simulink model "stmnucleo_I2C_temp_extendedMode"  (R2022a)
settings: Solver=FixedStepAuto  StartTime=0.0  StopTime=30  RelTol=1e-3  EnableMultiTasking=on
libraries: hdlsllib x4, simulink x4, mbedblockslib x4
settings Model: SimulationMode=external  ExtModeTrigDuration=10  Creator=The MathWorks, Inc.  LastModifiedBy=FUGAZI
settings SolverCC: AlgebraicLoopSolver=TrustRegion  MaxZcPerStep=1
settings DataIOCC: LimitDataPoints=on  ReturnWorkspaceOutputs=off
settings OptimizationCC: BlockReduction=off  LifeSpan=Inf  MaxStackSize=64
settings DebuggingCC: UnconnectedInputMsg=warning  UnconnectedOutputMsg=warning  UnconnectedLineMsg=warning  AllowSymbolicDim=off  SFUnexpectedBacktrackingDiag=warning  SFNoUnconditionalDefaultTransitionDiag=warning  SFExecutionAtInitializationDiag=none  SFMachineParentedDataDiag=warning  ArithmeticOperatorsInVariantConditions=warning
settings HardwareCC: ProdBitPerPointer=32  ProdBitPerSizeT=32  ProdBitPerPtrDiffT=32  ProdLargestAtomicInteger=Long  ProdLargestAtomicFloat=Double  ProdWordSize=32  ProdLongLongMode=on  ProdHWDeviceType=ARM Compatible->ARM Cortex
settings ModelReferenceCC: PropagateSignalLabelsOutOfModel=off
settings SFSimCC: SimUseLocalCustomCode=off
settings RTWCC: SystemTargetFile=ert.tlc  HardwareBoard=STM32 Nucleo L476RG  TemplateMakefile=ert_default_tmf  RTWUseLocalCustomCode=off  Toolchain=GNU Tools for ARM Embedded Processors  BuildConfiguration=Faster Runs  DLArmComputeVersion=19.05
settings CodeAppCC: StateflowObjectComments=on
settings ERTTargetCC: CodeReplacementLibrary=ARM Cortex-M (Optimized)  MultiwordLength=2048  ERTCustomFileBanners=off  SupportContinuousTime=on  SupportNonInlinedSFcns=on  RemoveResetFunc=off  ModelStepFunctionPrototypeControlCompliant=off  ExtModeTransport=3  ExtModeStaticAlloc=on  ExtModeStaticAllocSize=2000  ExtModeMexFile=ext_xcp  ExtModeIntrfLevel=Level2 - Open  ConvertIfToSwitch=off  SuppressUnreachableDefaultCases=off
settings ConfigComp: CovMetricSettings=dw  CovSaveCumulativeToWorkspaceVar=on  CovSaveSingleToWorkspaceVar=on  CovExternalEMLEnable=off

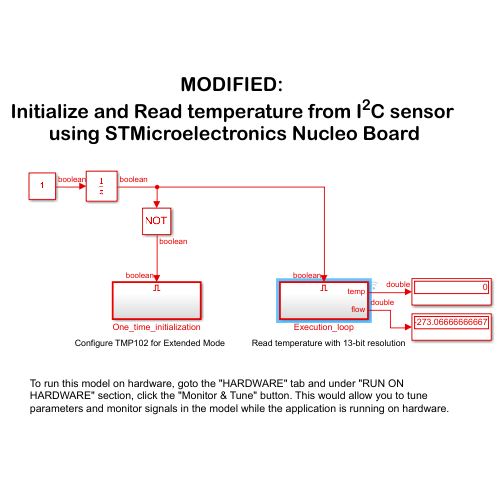
[thumbnail: Simulink's stored preview of the top-level diagram]
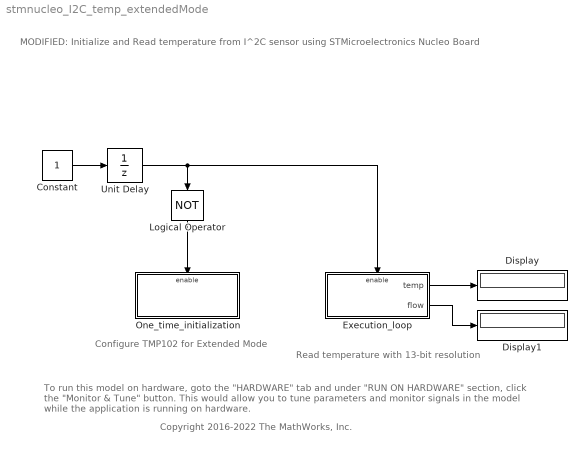
== system stmnucleo_I2C_temp_extendedMode ==
  note: Read temperature with 13-bit resolution
  note: Configure TMP102 for Extended Mode
  note: Copyright 2016-2022 The MathWorks, Inc.
  note: MODIFIED:
      | Initialize and Read temperature from I^2C sensor
      |  using STMicroelectronics Nucleo Board
  note: To run this model on hardware, goto the "HARDWARE" tab and under "RUN ON HARDWARE" section, click the "Monitor & Tune" button. This would allow you to tune parameters and monitor signals in the model while the application is running on hardware.
  Constant : Constant  OutDataTypeStr=boolean  SampleTime=0.1
  Display : Display
      settings: Format=hex (Stored Integer)
  Display1 : Display
      settings: Format=hex (Stored Integer)
  Execution_loop : Subsystem  TreatAsAtomicUnit=on
  Logical Operator : Logic  Operator=NOT  AllPortsSameDT=off  OutDataTypeStr=boolean
  One_time_initialization : Subsystem  TreatAsAtomicUnit=on
  Unit Delay : UnitDelay  SampleTime=-1  HasFrameUpgradeWarning=on
  wires:
  Constant/1 -> Unit Delay/1
  Unit Delay/1 -> Execution_loop/Enable, Logical Operator/1
  Logical Operator/1 -> One_time_initialization/Enable
  Execution_loop/1(temp) -> Display/1
  Execution_loop/2(flow) -> Display1/1

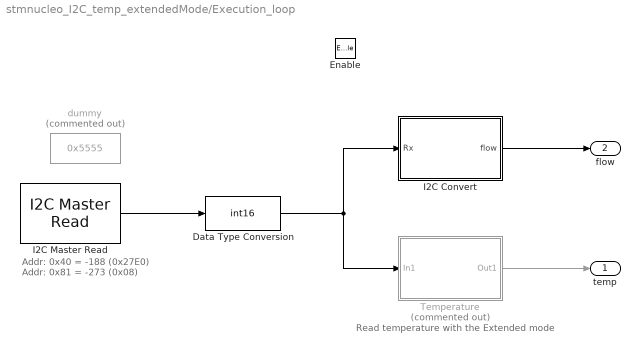
== system stmnucleo_I2C_temp_extendedMode/Execution_loop ==
  note: Addr: 0x40 = -188 (0x27E0)
      | Addr: 0x81 = -273 (0x08)
  note: Read temperature with the Extended mode
  Enable : EnablePort
  Data Type Conversion : DataTypeConversion  OutDataTypeStr=int16  ConvertRealWorld=Stored Integer (SI)  SaturateOnIntegerOverflow=off  RndMeth=Floor
  I2C Convert : Subsystem
  I2C Master Read : mbedblockslib/I2C Master Read  I2CModule=0  Mode=Master  SlaveAddress=hex2dec('40')  SlaveByteOrder=BigEndian  Direction=Receiver  RegisterAddressMode=on  RegisterAddress=uint8(0)  SlaveDataType=uint16  DataLength=1  NoAck=off  RepeatedStart=off  OutputStatus=off  SampleTime=0.1
      settings: SourceProductBaseCode=MICROBIT,NUCLEO,STMICRODIS
  Temperature : Subsystem  Commented=on
  dummy : Constant  Commented=on  Value=0x5555
  temp : Outport  InitialOutput=0  VectorParamsAs1DForOutWhenUnconnected=off
  flow : Outport  Port=2  InitialOutput=0  VectorParamsAs1DForOutWhenUnconnected=off
  wires:
  Data Type Conversion/1 -> Temperature/1(In1), I2C Convert/1(Rx)
  Temperature/1(Out1) -> temp/1
  I2C Convert/1(flow) -> flow/1
  I2C Master Read/1 -> Data Type Conversion/1

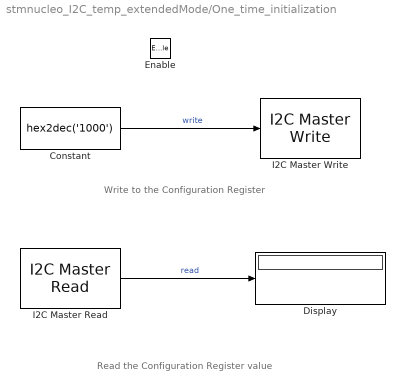
== system stmnucleo_I2C_temp_extendedMode/One_time_initialization ==
  note: Write to the Configuration Register
  note: Read the Configuration Register value
  Enable : EnablePort
  Constant : Constant  Value=hex2dec('1000')  OutDataTypeStr=uint16
  Display : Display
      settings: Format=hex (Stored Integer)
  I2C Master Read : mbedblockslib/I2C Master Read  I2CModule=0  Mode=Master  SlaveAddress=hex2dec('40')  SlaveByteOrder=BigEndian  Direction=Receiver  RegisterAddressMode=on  RegisterAddress=uint8(1)  SlaveDataType=uint16  DataLength=1  NoAck=off  RepeatedStart=off  OutputStatus=off  SampleTime=0.1
      settings: SourceProductBaseCode=MICROBIT,NUCLEO,STMICRODIS
  I2C Master Write : mbedblockslib/I2C Master Write  I2CModule=0  Mode=Master  SlaveAddress=hex2dec('40')  SlaveByteOrder=BigEndian  Direction=Transmitter  RegisterAddressMode=on  RegisterAddress=uint8(1)  SlaveDataType=uint8  DataLength=2  NoAck=off  RepeatedStart=off  OutputStatus=off
      settings: SourceProductBaseCode=MICROBIT,NUCLEO,STMICRODIS
  wires:
  Constant/1 -> I2C Master Write/1  "write"
  I2C Master Read/1 -> Display/1  "read"

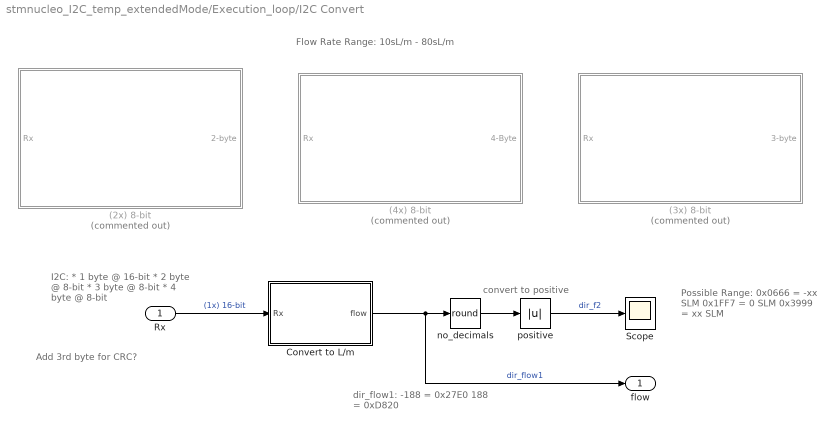
== system stmnucleo_I2C_temp_extendedMode/Execution_loop/I2C Convert ==
  note: dir_flow1:
      | -188 = 0x27E0
      | 188 = 0xD820
  note: Possible Range:
      | 0x0666 = -xx SLM
      | 0x1FF7 = 0 SLM
      | 0x3999 = xx SLM
  note: Flow Rate Range: 10sL/m - 80sL/m
  note: I2C:
      | * 1 byte @ 16-bit
      | * 2 byte @ 8-bit
      | * 3 byte @ 8-bit
      | * 4 byte @ 8-bit
  note: Add 3rd byte for CRC?
  note: convert to positive
  Rx : Inport
  (2x) 8-bit : Subsystem  Commented=on
  (3x) 8-bit : Subsystem  Commented=on
  (4x) 8-bit : Subsystem  Commented=on
  Convert to L/m : Subsystem
  Scope : Scope
  no_decimals : Rounding  Operator=round
  positive : Abs  SaturateOnIntegerOverflow=off
  flow : Outport
  wires:
  Convert to L/m/1(flow) -> flow/1, no_decimals/1  "dir_flow1"
  no_decimals/1 -> positive/1
  Rx/1 -> Convert to L/m/1(Rx)  "(1x) 16-bit"
  positive/1 -> Scope/1  "dir_f2"

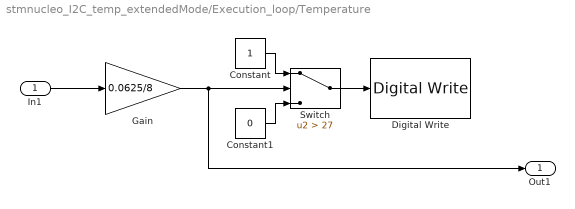
== system stmnucleo_I2C_temp_extendedMode/Execution_loop/Temperature ==
  In1 : Inport
  Constant : Constant  OutDataTypeStr=uint8
  Constant1 : Constant  Value=0  OutDataTypeStr=uint8
  Digital Write : mbedblockslib/Digital Write  Pin=D13  Direction=output
      settings: SourceProductBaseCode=MICROBIT,NUCLEO,STMICRODIS
  Gain : Gain  Gain=0.0625/8  OutDataTypeStr=single
  Switch : Switch  Criteria=u2 > Threshold  Threshold=27  SaturateOnIntegerOverflow=off  InputSameDT=off
  Out1 : Outport
  wires:
  Constant/1 -> Switch/1
  Constant1/1 -> Switch/3
  Gain/1 -> Out1/1, Switch/2
  In1/1 -> Gain/1
  Switch/1 -> Digital Write/1

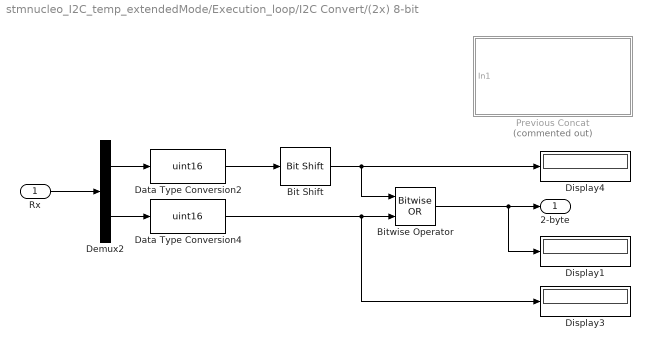
== system stmnucleo_I2C_temp_extendedMode/Execution_loop/I2C Convert/(2x) 8-bit ==
  Rx : Inport
  Bit Shift : hdlsllib/Logic and Bit Operations/Bit Shift  mode=Shift Left Logical  N=8
  Bitwise Operator : simulink/Logic and Bit Operations/Bitwise Operator  logicop=OR  UseBitMask=off  NumInputPorts=2  BitMask=bin2dec('11011001')  BitMaskRealWorld=Stored Integer
  Data Type Conversion2 : DataTypeConversion  OutDataTypeStr=uint16  SaturateOnIntegerOverflow=off  RndMeth=Floor
  Data Type Conversion4 : DataTypeConversion  OutDataTypeStr=uint16  SaturateOnIntegerOverflow=off  RndMeth=Floor
  Demux2 : Demux  Outputs=2
  Display1 : Display
      settings: Format=hex (Stored Integer)
  Display3 : Display
      settings: Format=hex (Stored Integer)
  Display4 : Display
      settings: Format=hex (Stored Integer)
  Previous Concat : Subsystem  Commented=on
  2-byte : Outport
  wires:
  Rx/1 -> Demux2/1
  Demux2/1 -> Data Type Conversion2/1
  Data Type Conversion2/1 -> Bit Shift/1
  Bit Shift/1 -> Display4/1, Bitwise Operator/1
  Data Type Conversion4/1 -> Display3/1, Bitwise Operator/2
  Demux2/2 -> Data Type Conversion4/1
  Bitwise Operator/1 -> Display1/1, 2-byte/1

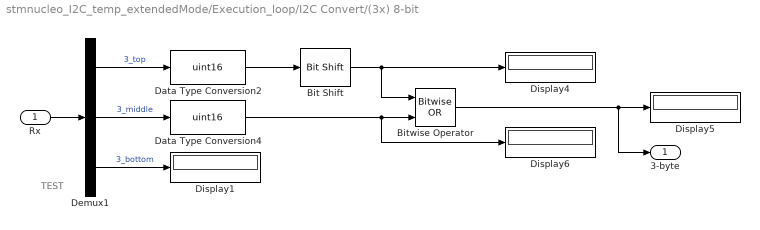
== system stmnucleo_I2C_temp_extendedMode/Execution_loop/I2C Convert/(3x) 8-bit ==
  note: TEST
  Rx : Inport
  Bit Shift : hdlsllib/Logic and Bit Operations/Bit Shift  mode=Shift Left Logical  N=8
  Bitwise Operator : simulink/Logic and Bit Operations/Bitwise Operator  logicop=OR  UseBitMask=off  NumInputPorts=2  BitMask=bin2dec('11011001')  BitMaskRealWorld=Stored Integer
  Data Type Conversion2 : DataTypeConversion  OutDataTypeStr=uint16  SaturateOnIntegerOverflow=off  RndMeth=Floor
  Data Type Conversion4 : DataTypeConversion  OutDataTypeStr=uint16  SaturateOnIntegerOverflow=off  RndMeth=Floor
  Demux1 : Demux  Outputs=3
  Display{1,4..6} (4 alike) : Display
      settings: Format=hex (Stored Integer)
  3-byte : Outport
  wires:
  Bit Shift/1 -> Bitwise Operator/1, Display4/1
  Data Type Conversion4/1 -> Display6/1, Bitwise Operator/2
  Bitwise Operator/1 -> 3-byte/1, Display5/1
  Data Type Conversion2/1 -> Bit Shift/1
  Rx/1 -> Demux1/1
  Demux1/1 -> Data Type Conversion2/1  "3_top"
  Demux1/2 -> Data Type Conversion4/1  "3_middle"
  Demux1/3 -> Display1/1  "3_bottom"

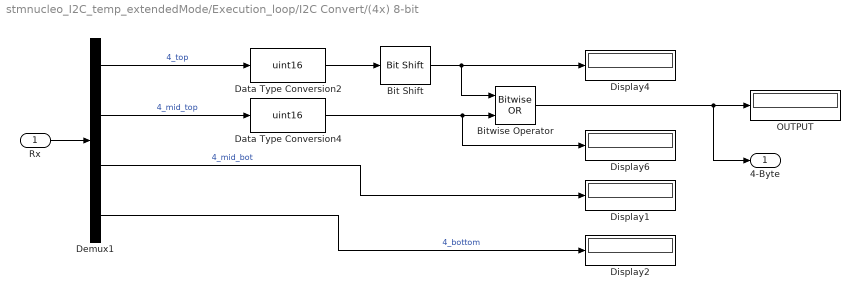
== system stmnucleo_I2C_temp_extendedMode/Execution_loop/I2C Convert/(4x) 8-bit ==
  Rx : Inport
  Bit Shift : hdlsllib/Logic and Bit Operations/Bit Shift  mode=Shift Left Logical  N=8
  Bitwise Operator : simulink/Logic and Bit Operations/Bitwise Operator  logicop=OR  UseBitMask=off  NumInputPorts=2  BitMask=bin2dec('11011001')  BitMaskRealWorld=Stored Integer
  Data Type Conversion2 : DataTypeConversion  OutDataTypeStr=uint16  SaturateOnIntegerOverflow=off  RndMeth=Floor
  Data Type Conversion4 : DataTypeConversion  OutDataTypeStr=uint16  SaturateOnIntegerOverflow=off  RndMeth=Floor
  Demux1 : Demux
  Display{1..2,4,6} (4 alike) : Display
      settings: Format=hex (Stored Integer)
  OUTPUT : Display
      settings: Format=hex (Stored Integer)
  4-Byte : Outport
  wires:
  Data Type Conversion2/1 -> Bit Shift/1
  Bitwise Operator/1 -> 4-Byte/1, OUTPUT/1
  Bit Shift/1 -> Display4/1, Bitwise Operator/1
  Demux1/4 -> Display2/1  "4_bottom"
  Rx/1 -> Demux1/1
  Demux1/2 -> Data Type Conversion4/1  "4_mid_top"
  Demux1/1 -> Data Type Conversion2/1  "4_top"
  Data Type Conversion4/1 -> Display6/1, Bitwise Operator/2
  Demux1/3 -> Display1/1  "4_mid_bot"

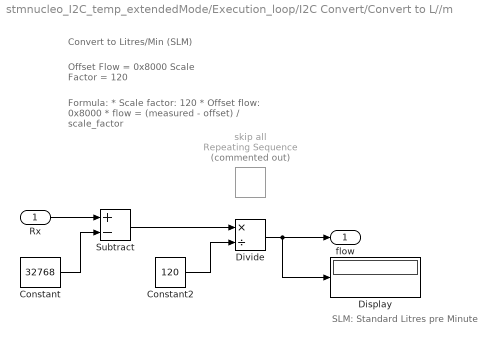
== system stmnucleo_I2C_temp_extendedMode/Execution_loop/I2C Convert/Convert to L//m ==
  note: SLM: Standard Litres pre Minute
  note: Convert to Litres/Min (SLM)
  note: Offset Flow = 0x8000
      | Scale Factor = 120
  note: Formula:
      | * Scale factor: 120
      | * Offset flow: 0x8000
      | * flow = (measured - offset) / scale_factor
  Rx : Inport
  Constant : Constant  Value=32768
  Constant2 : Constant  Value=120
  Display : Display
  Divide : Product  Inputs=*/
  Subtract : Sum  Inputs=+-
  skip all : simulink/Sources/Repeating Sequence  Commented=on  rep_seq_t=[0 1.3 1.31 2.5 2.51]  rep_seq_y=[30 30 150 150 30]
  flow : Outport
  wires:
  Divide/1 -> Display/1, flow/1
  Subtract/1 -> Divide/1
  Constant2/1 -> Divide/2
  Constant/1 -> Subtract/2
  Rx/1 -> Subtract/1

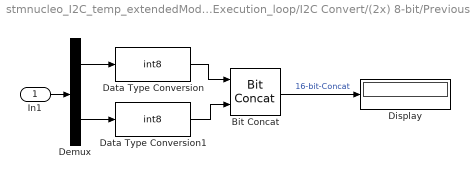
== system stmnucleo_I2C_temp_extendedMode/Execution_loop/I2C Convert/(2x) 8-bit/Previous Concat ==
  In1 : Inport
  Bit Concat : hdlsllib/Logic and Bit Operations/Bit Concat  numInputs=2
  Data Type Conversion : DataTypeConversion  OutDataTypeStr=int8  SaturateOnIntegerOverflow=off  RndMeth=Floor
  Data Type Conversion1 : DataTypeConversion  OutDataTypeStr=int8  SaturateOnIntegerOverflow=off  RndMeth=Floor
  Demux : Demux  Outputs=2
  Display : Display
      settings: Format=hex (Stored Integer)
  wires:
  Data Type Conversion/1 -> Bit Concat/1
  Bit Concat/1 -> Display/1  "16-bit-Concat"
  Demux/2 -> Data Type Conversion1/1
  Data Type Conversion1/1 -> Bit Concat/2
  Demux/1 -> Data Type Conversion/1
  In1/1 -> Demux/1
